simulink model "part2_1"  (R2023b)
settings: Solver=VariableStepAuto  StartTime=0.0  StopTime=10.0  MaxStep=0.01  RelTol=1e-3
settings Model: Creator=82354
settings SolverCC: AlgebraicLoopSolver=TrustRegion
settings DataIOCC: ReturnWorkspaceOutputs=off
settings DebuggingCC: UnconnectedInputMsg=warning  UnconnectedOutputMsg=warning  UnconnectedLineMsg=warning  ArithmeticOperatorsInVariantConditions=warning
settings ModelReferenceCC: EnableRefExpFcnMdlSchedulingChecks=on
settings SFSimCC: SimUseLocalCustomCode=off  CustomCodeUndefinedFunction=UseInterfaceOnly
settings RTWCC: RTWUseLocalCustomCode=off

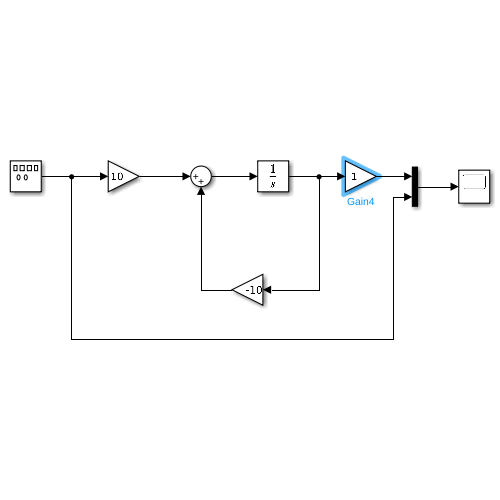
[thumbnail: Simulink's stored preview of the top-level diagram]
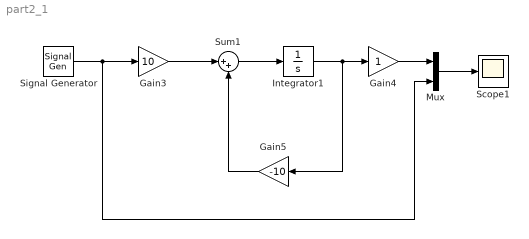
== system part2_1 ==
  Gain3 : Gain  Gain=10
  Gain4 : Gain
  Gain5 : Gain  Gain=-10
  Integrator1 : Integrator  InitialCondition=1
  Mux : Mux  Inputs=2
  Scope1 : Scope
  Signal Generator : SignalGenerator  Amplitude=0  Frequency=0.1  Units=rad/sec
  Sum1 : Sum  Inputs=|++
  wires:
  Integrator1/1 -> Gain5/1, Gain4/1
  Gain3/1 -> Sum1/1
  Sum1/1 -> Integrator1/1
  Gain5/1 -> Sum1/2
  Gain4/1 -> Mux/1
  Mux/1 -> Scope1/1
  Signal Generator/1 -> Mux/2, Gain3/1
